simulink model "Gorev3"  (R2019b)
settings: Solver=ode45  StartTime=0.0  StopTime=10.0  RelTol=1e-3
libraries: simulink x1
settings Model: Creator=Bekircan Keceoglu  LastModifiedBy=Bekircan Keceoglu

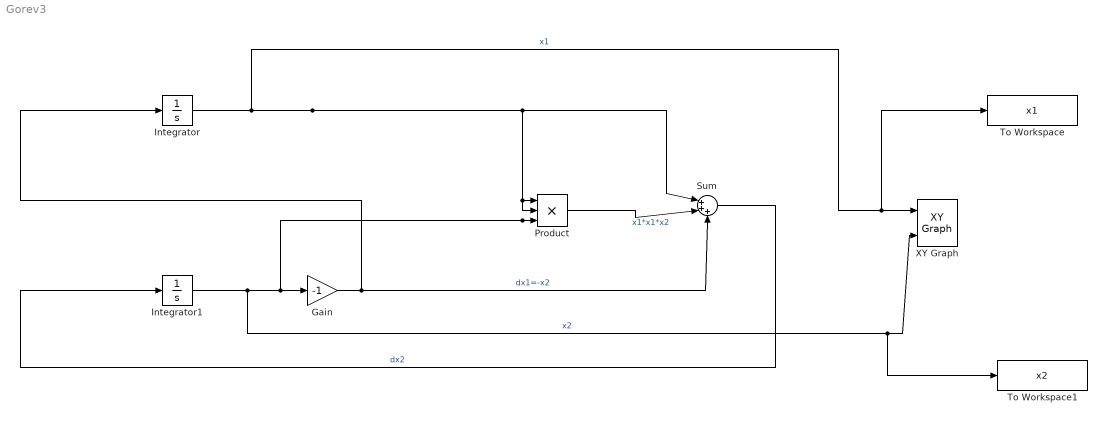
== system Gorev3 ==
  Gain : Gain  Gain=-1
  Integrator : Integrator  InitialCondition=1
  Integrator1 : Integrator  InitialCondition=1
  Product : Product  Inputs=3
  Sum : Sum  Inputs=|+++
  To Workspace : ToWorkspace  VariableName=x1  SampleTime=-1
  To Workspace1 : ToWorkspace  VariableName=x2  SampleTime=-1
  XY Graph : simulink/Sinks/XY Graph  xmin=-0.6  xmax=1.1  ymin=-0.4  ymax=1.2  st=-1
  wires:
  Gain/1 -> Sum/3, Integrator/1  "dx1=-x2"
  Sum/1 -> Integrator1/1  "dx2"
  Integrator/1 -> To Workspace/1, XY Graph/1, Product/2, Product/1, Sum/1  "x1"
  Integrator1/1 -> To Workspace1/1, XY Graph/2, Product/3, Gain/1  "x2"
  Product/1 -> Sum/2  "x1*x1*x2"
